simulink model "Quadcopter_sim1"  (R2021a)
settings: Solver=VariableStepAuto  StartTime=0.0  StopTime=t_stop  RelTol=1e-3
values from neighbouring files (symbols this model uses):
  b = 0.001    [Exercise2.m]    (also in Exercise2_3.m)
  g = 9.81    [Exercise2.m]    (also in Exercise2_3.m)
  Ixx = 3e-06    [Exercise2.m]    (also in Exercise2_3.m)
  Iyy = 3e-06    [Exercise2.m]    (also in Exercise2_3.m)
  Izz = 1e-05    [Exercise2.m]    (also in Exercise2_3.m)
  k = 0.01    [Exercise2.m]    (also in Exercise2_3.m)
  L = 0.225    [Exercise2.m]    (also in Exercise2_3.m)
  m = 0.5    [Exercise2.m]    (also in Exercise2_3.m)
  omega1 = 10000    [Exercise2_3.m]
  omega2 = 0    [Exercise2_3.m]
  omega3 = 10000    [Exercise2_3.m]
  omega4 = 0    [Exercise2_3.m]
settings Model: Creator=emilm  LastModifiedBy=emilm

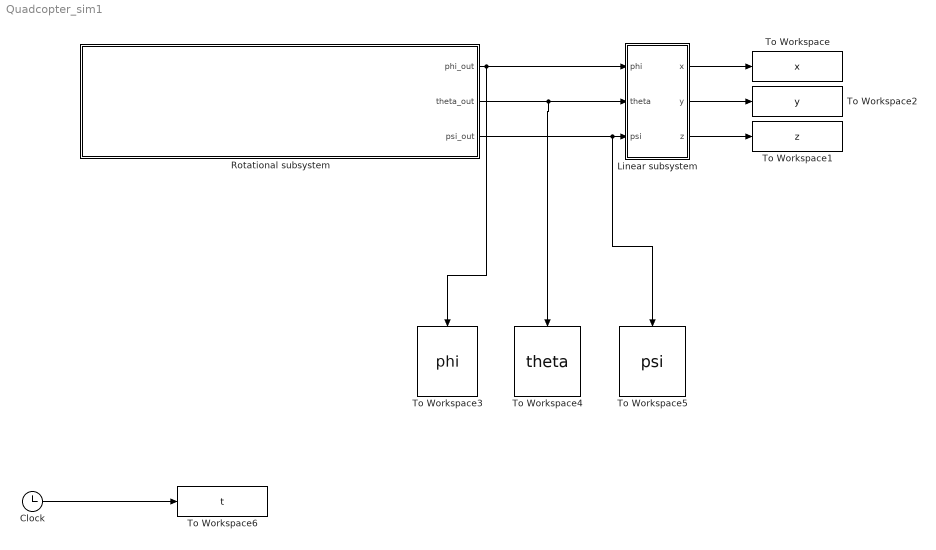
== system Quadcopter_sim1 ==
  Clock : Clock
  Linear subsystem : Subsystem
  Rotational subsystem : Subsystem
  To Workspace : ToWorkspace  VariableName=x  SampleTime=-1
  To Workspace1 : ToWorkspace  VariableName=z  SampleTime=-1
  To Workspace2 : ToWorkspace  VariableName=y  SampleTime=-1
  To Workspace3 : ToWorkspace  VariableName=phi  SampleTime=-1
  To Workspace4 : ToWorkspace  VariableName=theta  SampleTime=-1
  To Workspace5 : ToWorkspace  VariableName=psi  SampleTime=-1
  To Workspace6 : ToWorkspace  VariableName=t  SampleTime=-1
  wires:
  Rotational subsystem/1(phi_out) -> Linear subsystem/1(phi), To Workspace3/1
  Rotational subsystem/2(theta_out) -> To Workspace4/1, Linear subsystem/2(theta)
  Rotational subsystem/3(psi_out) -> To Workspace5/1, Linear subsystem/3(psi)
  Linear subsystem/1(x) -> To Workspace/1
  Linear subsystem/2(y) -> To Workspace2/1
  Linear subsystem/3(z) -> To Workspace1/1
  Clock/1 -> To Workspace6/1

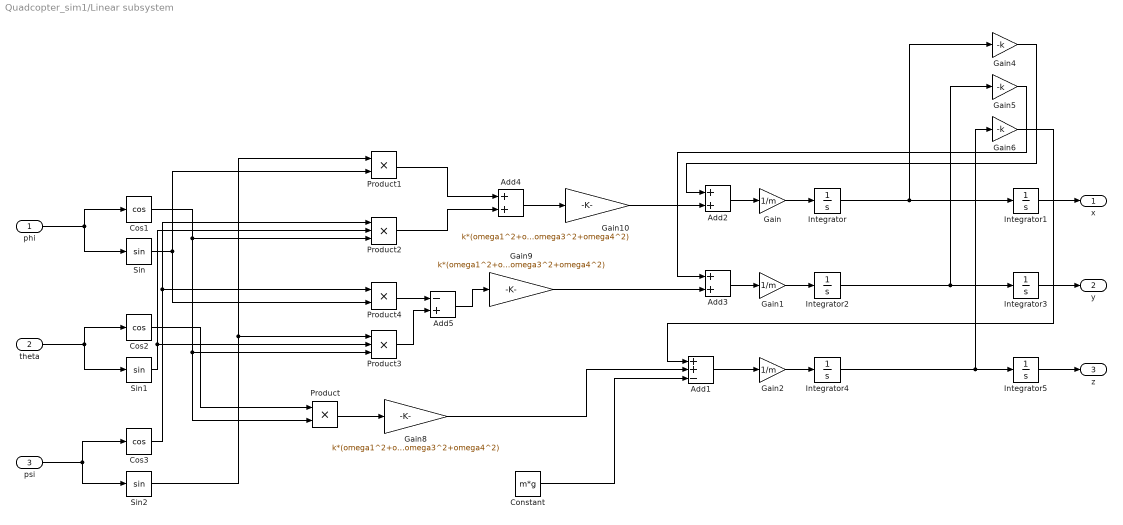
== system Quadcopter_sim1/Linear subsystem ==
  phi : Inport
  theta : Inport  Port=2
  psi : Inport  Port=3
  Add1 : Sum  Inputs=++-
  Add2 : Sum
  Add3 : Sum
  Add4 : Sum
  Add5 : Sum  Inputs=-+
  Constant : Constant  Value=m*g
  Cos1 : Trigonometry  Operator=cos
  Cos2 : Trigonometry  Operator=cos
  Cos3 : Trigonometry  Operator=cos
  Gain : Gain  Gain=1/m
  Gain1 : Gain  Gain=1/m
  Gain10 : Gain  Gain=k*(omega1^2+omega2^2+omega3^2+omega4^2)
  Gain2 : Gain  Gain=1/m
  Gain4 : Gain  Gain=-k
  Gain5 : Gain  Gain=-k
  Gain6 : Gain  Gain=-k
  Gain8 : Gain  Gain=k*(omega1^2+omega2^2+omega3^2+omega4^2)
  Gain9 : Gain  Gain=k*(omega1^2+omega2^2+omega3^2+omega4^2)
  Integrator{,1..5} (6 alike) : Integrator
  Product : Product
  Product1 : Product
  Product2 : Product  Inputs=3
  Product3 : Product  Inputs=3
  Product4 : Product
  Sin : Trigonometry
  Sin1 : Trigonometry
  Sin2 : Trigonometry
  x : Outport
  y : Outport  Port=2
  z : Outport  Port=3
  wires:
  Gain4/1 -> Add2/1
  Gain1/1 -> Integrator2/1
  Gain6/1 -> Add1/1
  Add2/1 -> Gain/1
  Gain5/1 -> Add3/1
  Integrator5/1 -> z/1
  Gain/1 -> Integrator/1
  Integrator2/1 -> Gain5/1, Integrator3/1
  Gain2/1 -> Integrator4/1
  Integrator4/1 -> Gain6/1, Integrator5/1
  Add3/1 -> Gain1/1
  Gain9/1 -> Add3/2
  Gain8/1 -> Add1/2
  Gain10/1 -> Add2/2
  Integrator/1 -> Gain4/1, Integrator1/1
  Add1/1 -> Gain2/1
  Integrator1/1 -> x/1
  Integrator3/1 -> y/1
  Product/1 -> Gain8/1
  phi/1 -> Sin/1, Cos1/1
  theta/1 -> Sin1/1, Cos2/1
  psi/1 -> Sin2/1, Cos3/1
  Cos2/1 -> Product/1
  Cos1/1 -> Product3/3, Product/2, Product2/3
  Constant/1 -> Add1/3
  Add4/1 -> Gain10/1
  Product1/1 -> Add4/1
  Product2/1 -> Add4/2
  Sin2/1 -> Product3/1, Product1/1
  Sin/1 -> Product1/2, Product4/2
  Cos3/1 -> Product4/1, Product2/1
  Sin1/1 -> Product3/2, Product2/2
  Add5/1 -> Gain9/1
  Product4/1 -> Add5/1
  Product3/1 -> Add5/2

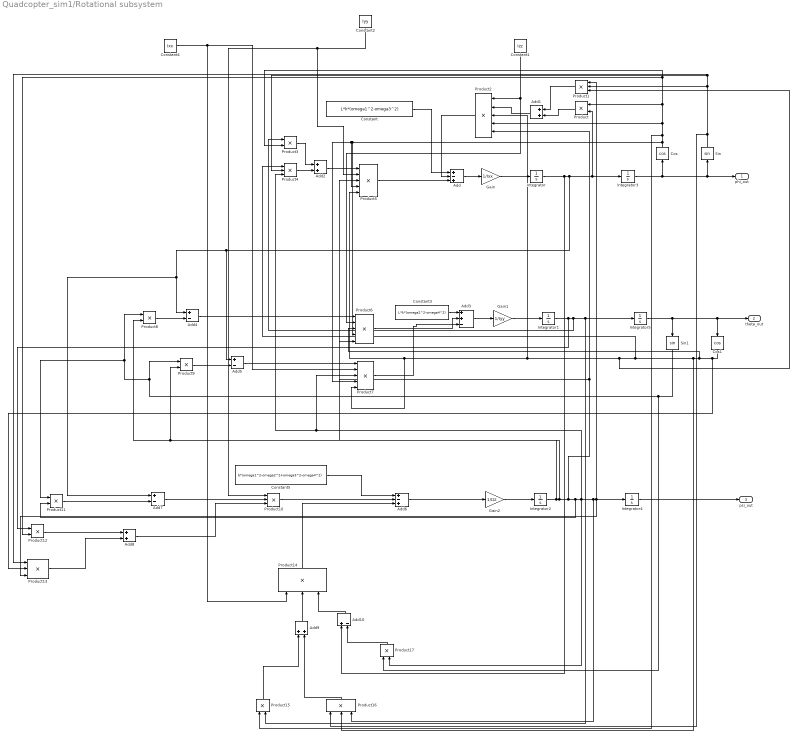
== system Quadcopter_sim1/Rotational subsystem ==
  Add : Sum  Inputs=+-+
  Add{1..2,8..9} (4 alike) : Sum
  Add{4..5,7,10} (4 alike) : Sum  Inputs=+-
  Add3 : Sum  Inputs=++-
  Add6 : Sum  Inputs=+-+
  Constant : Constant  Value=L*k*(omega1^2-omega3^2)
  Constant1 : Constant  Value=Izz
  Constant2 : Constant  Value=Iyy
  Constant3 : Constant  Value=L*k*(omega2^2-omega4^2)
  Constant4 : Constant  Value=Ixx
  Constant5 : Constant  Value=b*(omega1^2-omega2^2+omega3^2-omega4^2)
  Cos : Trigonometry  Operator=cos
  Cos1 : Trigonometry  Operator=cos
  Gain : Gain  Gain=1/Ixx
  Gain1 : Gain  Gain=1/Iyy
  Gain2 : Gain  Gain=1/Izz
  Integrator{,1..5} (6 alike) : Integrator
  Product{,3,8..9,11..12,15,17} (8 alike) : Product
  Product{1,4,10,13..14,16} (6 alike) : Product  Inputs=3
  Product{2,5..7} (4 alike) : Product  Inputs=5
  Sin : Trigonometry
  Sin1 : Trigonometry
  phi_out : Outport
  theta_out : Outport  Port=2
  psi_out : Outport  Port=3
  wires:
  Gain1/1 -> Integrator1/1
  Gain/1 -> Integrator/1
  Gain2/1 -> Integrator2/1
  Integrator/1 -> Add10/1, Add5/1, Add4/1, Add7/1, Product/2, Integrator3/1
  Integrator1/1 -> Product12/1, Product3/1, Product15/2, Integrator5/1
  Integrator2/1 -> Product6/5, Product9/2, Product8/2, Product5/3, Product2/5, Product11/2, Product17/2, Product7/3, Product4/3, Product16/3, Product13/3, Product1/1, Integrator4/1
  Integrator3/1 -> Cos/1, Sin/1, phi_out/1
  Integrator5/1 -> Sin1/1, Cos1/1, theta_out/1
  Integrator4/1 -> psi_out/1
  Add/1 -> Gain/1
  Constant/1 -> Add/1
  Cos/1 -> Product7/4, Product5/4, Product6/4, Product15/1, Product12/2, Product3/2, Product/1, Product2/4
  Product/1 -> Add1/2
  Product1/1 -> Add1/1
  Cos1/1 -> Product16/2, Product5/5, Product7/5, Product2/3, Product1/3, Product4/1, Product6/3, Product13/2
  Sin/1 -> Product16/1, Product13/1, Product4/2, Product1/2
  Constant1/1 -> Product6/2, Product2/1
  Add1/1 -> Product2/2
  Product2/1 -> Add/2
  Product4/1 -> Add2/2
  Product3/1 -> Add2/1
  Product5/1 -> Add/3
  Add2/1 -> Product5/1
  Constant2/1 -> Product10/1, Product5/2
  Constant3/1 -> Add3/1
  Add3/1 -> Gain1/1
  Product6/1 -> Add3/2
  Product7/1 -> Add3/3
  Add4/1 -> Product6/1
  Product8/1 -> Add4/2
  Sin1/1 -> Product17/1, Product9/1, Product11/1, Product8/1
  Add5/1 -> Product7/1
  Product9/1 -> Add5/2
  Constant4/1 -> Product14/1, Product7/2
  Add6/1 -> Gain2/1
  Constant5/1 -> Add6/1
  Product10/1 -> Add6/2
  Add7/1 -> Product10/2
  Product11/1 -> Add7/2
  Add8/1 -> Product10/3
  Product12/1 -> Add8/1
  Product13/1 -> Add8/2
  Product14/1 -> Add6/3
  Add9/1 -> Product14/2
  Product16/1 -> Add9/2
  Product15/1 -> Add9/1
  Add10/1 -> Product14/3
  Product17/1 -> Add10/2
